simulink model "bikeBBR"  (Simulink 6.1)
settings: Solver=ode23s  StartTime=0.0  StopTime=50  RelTol=1e-3
values from neighbouring files (symbols this model uses):
  ABBR = [0 8.39044421109 0 8.09876894767 1 -0.112133410006 0 6.81426106958 0 -17.7563110842 0 -7.30629683726 ... (16 elements, 4x4)]    [BBR.mat]
  BBBR = [0  0; 0.0105572020466  -0.0498370711137; 0  0; -0.0498370711137  3.02856047537]    [BBR.mat]
  CBBR = [1 0 0 0 0 1 0 0 0 0 1 0 ... (16 elements, 4x4)]    [BBR.mat]
  DBBR = [0  0; 0  0; 0  0; 0  0]    [BBR.mat]
  kagress = 1    [BBR.mat]
  v = 5    [BBR.mat]
libraries: simulink x6
settings Model: LastModifiedBy=hess
settings OptimizationCC: InlineParams=on
settings DebuggingCC: SolverPrmCheckMsg=warning

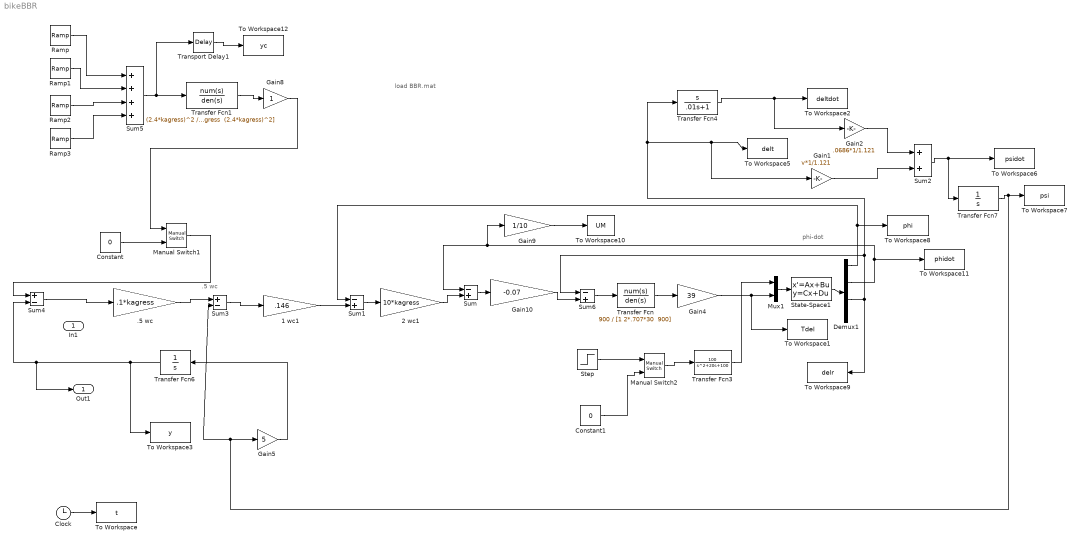
== system bikeBBR ==
  note: phi-dot
  note: .5 wc
  note: load BBR.mat
  In1 : Inport  Port=1  LatchInput=off
  .5 wc : Gain  Gain=.1*kagress
  1 wc1 : Gain  Gain=.146
  2 wc1 : Gain  Gain=10*kagress
  Clock : Clock
      settings: Decimation=10
  Constant : Constant  Value=0
  Constant1 : Constant  Value=0
  Demux1 : Demux
  Gain1 : Gain  Gain=v*1/1.121
  Gain10 : Gain  Gain=-0.07
  Gain2 : Gain  Gain=.0686*1/1.121
  Gain4 : Gain  Gain=39
  Gain5 : Gain  Gain=5
  Gain8 : Gain
  Gain9 : Gain  Gain=1/10
  Manual Switch1 : simulink/Signal Routing/Manual Switch  sw=1  action=0
  Manual Switch2 : simulink/Signal Routing/Manual Switch  sw=0  action=0
  Mux1 : Mux  Inputs=2
  Ramp : simulink/Sources/Ramp  slope=1  start=7  X0=0
  Ramp1 : simulink/Sources/Ramp  slope=-1  start=9  X0=0
  Ramp2 : simulink/Sources/Ramp  slope=-1  start=17  X0=0
  Ramp3 : simulink/Sources/Ramp  slope=1  start=19  X0=0
  State-Space1 : StateSpace  A=ABBR  B=BBBR  C=CBBR  D=DBBR
  Step : Step  Time=10  SampleTime=0
  Sum : Sum  Inputs=-+
  Sum1 : Sum  Inputs=-+
  Sum2 : Sum
  Sum3 : Sum  Inputs=+-
  Sum4 : Sum  Inputs=+-
  Sum5 : Sum  Inputs=++++
  Sum6 : Sum  Inputs=-+
  To Workspace : ToWorkspace  VariableName=t  SampleTime=-1  SaveFormat=Array
  To Workspace1 : ToWorkspace  VariableName=Tdel  SampleTime=-1  SaveFormat=Array
  To Workspace10 : ToWorkspace  VariableName=UM  SampleTime=-1  SaveFormat=Array
  To Workspace11 : ToWorkspace  VariableName=phidot  SampleTime=-1  SaveFormat=Array
  To Workspace12 : ToWorkspace  VariableName=yc  SampleTime=-1  SaveFormat=Array
  To Workspace2 : ToWorkspace  VariableName=deltdot  SampleTime=-1  SaveFormat=Array
  To Workspace3 : ToWorkspace  VariableName=y  SampleTime=-1  SaveFormat=Array
  To Workspace5 : ToWorkspace  VariableName=delt  SampleTime=-1  SaveFormat=Array
  To Workspace6 : ToWorkspace  VariableName=psidot  SampleTime=-1  SaveFormat=Array
  To Workspace7 : ToWorkspace  VariableName=psi  SampleTime=-1  SaveFormat=Array
  To Workspace8 : ToWorkspace  VariableName=phi  SampleTime=-1  SaveFormat=Array
  To Workspace9 : ToWorkspace  VariableName=delr  SampleTime=-1  SaveFormat=Array
  Transfer Fcn : TransferFcn  Numerator=900  Denominator="[1 2*.707*30  900]"
  Transfer Fcn1 : TransferFcn  Numerator=(2.4*kagress)^2  Denominator="[1 2*2.4*kagress  (2.4*kagress)^2]"
  Transfer Fcn3 : TransferFcn  Numerator=100  Denominator=[1 20 100]
  Transfer Fcn4 : TransferFcn  Numerator=[1 0]  Denominator=[.01 1]
  Transfer Fcn6 : TransferFcn  Orientation=left  Numerator=1  Denominator=[1 0]
  Transfer Fcn7 : TransferFcn  Numerator=1  Denominator=[1 0]
  Transport Delay1 : TransportDelay  DelayTime=3.05
  Out1 : Outport
  wires:
  Sum/1 -> Gain10/1
  Transfer Fcn4/1 -> To Workspace2/1, Gain2/1
  Gain2/1 -> Sum2/1
  Gain1/1 -> Sum2/2
  Sum2/1 -> Transfer Fcn7/1, To Workspace6/1
  Transfer Fcn7/1 -> To Workspace7/1, Gain5/1, Sum3/2
  Gain5/1 -> Transfer Fcn6/1
  Sum5/1 -> Transfer Fcn1/1, Transport Delay1/1
  Transfer Fcn6/1 -> To Workspace3/1, Sum4/2, Out1/1
  Constant/1 -> Manual Switch1/2
  Gain8/1 -> Manual Switch1/1
  Gain9/1 -> To Workspace10/1
  Clock/1 -> To Workspace/1
  Mux1/1 -> State-Space1/1
  State-Space1/1 -> Demux1/1
  Demux1/3 -> To Workspace9/1, Transfer Fcn4/1, To Workspace5/1, Gain1/1, Sum6/1
  Demux1/1 -> To Workspace8/1, Sum1/1
  Step/1 -> Manual Switch2/1
  Manual Switch2/1 -> Transfer Fcn3/1
  Constant1/1 -> Manual Switch2/2
  Demux1/2 -> To Workspace11/1, Gain9/1, Sum/1
  Ramp/1 -> Sum5/1
  Ramp1/1 -> Sum5/2
  Ramp2/1 -> Sum5/3
  Ramp3/1 -> Sum5/4
  Transfer Fcn/1 -> Gain4/1
  Transfer Fcn1/1 -> Gain8/1
  Sum6/1 -> Transfer Fcn/1
  Transport Delay1/1 -> To Workspace12/1
  Transfer Fcn3/1 -> Mux1/1
  Manual Switch1/1 -> Sum4/1
  1 wc1/1 -> Sum1/2
  Gain4/1 -> Mux1/2, To Workspace1/1
  Gain10/1 -> Sum6/2
  2 wc1/1 -> Sum/2
  Sum1/1 -> 2 wc1/1
  Sum3/1 -> 1 wc1/1
  .5 wc/1 -> Sum3/1
  Sum4/1 -> .5 wc/1
